simulink model "lab7_t8"  (R2021a)
settings: Solver=VariableStepAuto  StartTime=0.0  StopTime=10.0  RelTol=1e-3
settings Model: Creator=reemb  LastModifiedBy=reemb

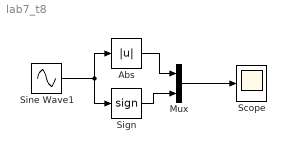
== system lab7_t8 ==
  Abs : Abs
  Mux : Mux  Inputs=2
  Scope : Scope
  Sign : Signum
  Sine Wave1 : Sin  SampleTime=0
  wires:
  Sign/1 -> Mux/2
  Sine Wave1/1 -> Sign/1, Abs/1
  Abs/1 -> Mux/1
  Mux/1 -> Scope/1
